simulink model "demo1"  (Simulink 10.0)
settings: Solver=VariableStepAuto  StartTime=0.0  StopTime=10.0  RelTol=1e-3
settings Model: Creator=unknownuser  LastModifiedBy=bhisma
settings DataIOCC: SaveFormat=Dataset  ReturnWorkspaceOutputs=on
settings OptimizationCC: LifeSpan=auto
settings DebuggingCC: UnderspecifiedInitializationDetection=Simplified  MergeDetectMultiDrivingBlocksExec=error  SFUnexpectedBacktrackingDiag=error  SFNoUnconditionalDefaultTransitionDiag=error  SFExecutionAtInitializationDiag=warning  ArithmeticOperatorsInVariantConditions=error
settings HardwareCC: ProdBitPerPointer=64  ProdBitPerSizeT=64  ProdBitPerPtrDiffT=64  ProdLargestAtomicFloat=Float  ProdIntDivRoundTo=Zero  ProdEndianess=LittleEndian  ProdWordSize=64  ProdHWDeviceType=Intel->x86-64 (Windows64)
settings ModelReferenceCC: PropagateSignalLabelsOutOfModel=on
settings SFSimCC: SimUseLocalCustomCode=on  CustomCodeUndefinedFunction=FilterOut
settings RTWCC: RTWUseLocalCustomCode=on
settings CodeAppCC: StateflowObjectComments=off
settings GRTTargetCC: TargetLangStandard=C99 (ISO)  CombineOutputUpdateFcns=on  GRTInterface=off
settings ConfigComp: CovMetricSettings=dwe  CovHtmlReporting=off  CovSaveCumulativeToWorkspaceVar=off  CovSaveSingleToWorkspaceVar=off

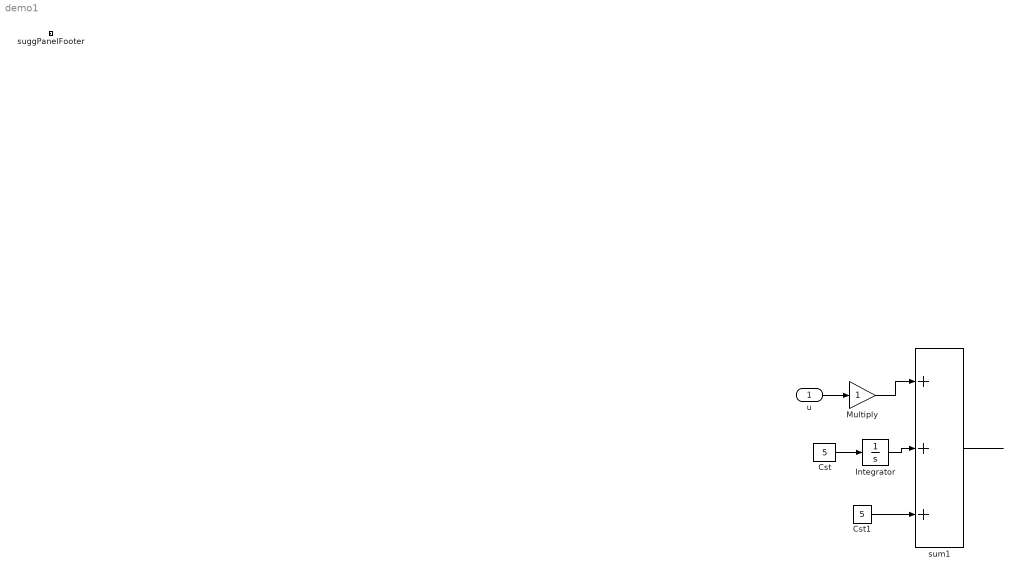
== system demo1 ==
  u : Inport
  Cst : Constant  Value=5
  Cst1 : Constant  Value=5
  Integrator : Integrator
  Multiply : Gain
  suggPanelFooter : Subsystem
      settings: OpenFcn=|
      | % callback function code for "Ignore Suggestions" button
      | 
      | state = getSharedVar('simvma_blockInsertionState');
      | 
      | % delete all suggested blocks
      | for i = 1 : length(state.suggs)
      |    sugg = state.suggs(i);
      |    try
      |        delete_block(sugg.blockPath);
      |    catch ME
      |    end
      | end
      | 
      | 
      | % delete all percentages
      | for i = 1 : length(state.percentTexts)
      |     percentText = state.percentTexts(i);
      |     percentTextPath = state.context.sud + "/" + percentText;
      |     try
      |         delete_block(percentTextPath);
      |     catch ME
      |     end
      | end
      | 
      | % unhighlightMrcbAndNeighbors(state.context, true);
      | 
      | % delete suggestion panel header
      | try
      |     delete_block(state.context.sud + "/suggPanelHeader");
      | catch ME
      | end
      | 
      | % delete suggestion panel body
      | try
      |     delete_block(state.context.sud + "/suggPanelBody");
      | catch ME
      | end
      | 
      | % - Unlike the header and the body, we are not able to delete the footer
      | %   subsystem (because we are in its own callback function)
      | % - To make it look like the subsystem is deleted, we set its size to a
      | %   point-size, and place it at the origin (away from any other blocks)
      | % - We delete this point-sized footer when "Simvma:Suggest Blocks" is called
      | %   next time (see dispBlkSuggsOnWorkspace.m)
      | 
      | footerPath = state.context.sud + "/suggPanelFooter";
      | set_param(footerPath, 'Position', [0 0 0 0]);
      | 
      | % reset the shared var simvma_blockInsertionState
      | setSharedVar('simvma_blockInsertionState', BlockInsertionState(NaN, NaN, NaN));
      | 
      | % % finally adjust zoom level
      | % set_param(blockInsertionState.context.sud, 'ZoomFactor', 'fit to view');
      mask Display: image('/Users/bhisma/courses/cse-700-simvma/simvma/images/sugg-panel-footer.png')
  sum1 : Sum  Inputs=+++  SaturateOnIntegerOverflow=on  InputSameDT=on  OutDataTypeStr=Inherit: Same as first input
  wires:
  Cst/1 -> Integrator/1
  sum1/1 -> ?
  Multiply/1 -> sum1/1
  Cst1/1 -> sum1/3
  Integrator/1 -> sum1/2
  u/1 -> Multiply/1

== system demo1/suggPanelFooter ==
